simulink model "Monitoring_R2017b"  (R2017b)
settings: Solver=FixedStepAuto  StartTime=0.0  StopTime=inf  FixedStep=0.01  RelTol=1e-3
undefined symbols (not defined in the file): f
libraries: aerolibanimutils x1, instrumentlib x1
settings Model: Creator=guilherme  LastModifiedBy=leona

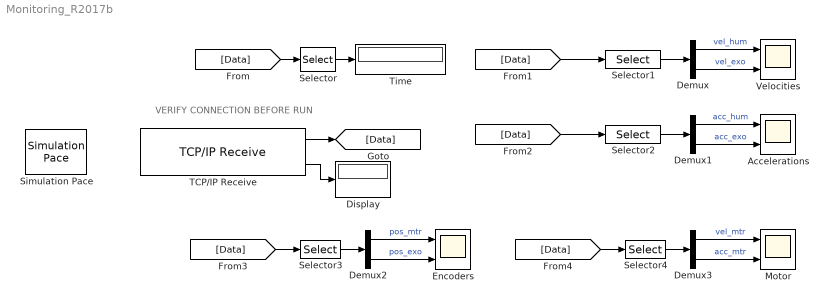
== system Monitoring_R2017b ==
  note: VERIFY CONNECTION BEFORE RUN
  Accelerations : Scope  NumInputPorts=2
  Demux{,1..3} (4 alike) : Demux  Outputs=2
  Display : Display
  Encoders : Scope  NumInputPorts=2
  Motor : Scope  NumInputPorts=2
  Selector : Selector  InputPortWidth=9  IndexOptions=Index vector (dialog)  Indices=[1]  OutputSizes=1
  Selector1 : Selector  InputPortWidth=9  IndexOptions=Index vector (dialog)  Indices=[2 3]  OutputSizes=1
  Selector2 : Selector  InputPortWidth=9  IndexOptions=Index vector (dialog)  Indices=[4 5]  OutputSizes=1
  Selector3 : Selector  InputPortWidth=9  IndexOptions=Index vector (dialog)  Indices=[6 7]  OutputSizes=1
  Selector4 : Selector  InputPortWidth=9  IndexOptions=Index vector (dialog)  Indices=[8 9]  OutputSizes=1
  Simulation Pace : aerolibanimutils/Simulation Pace  SimulationPace=1  SleepMode=Auto  OutputPaceError=off  SampleTime=-1
  TCP/IP Receive : instrumentlib/TCP//IP Receive  Host=0.0.0.0  Port=2324  DataSize="[1  9]"  EnableBlockingMode=off  Timeout=10  SampleTime=0.01  DataType=ASCII  ByteOrder=BigEndian  ASCIIFormatting=%f,%f,%f,%f,%f,%f,%f,%f,%f  Terminator=LF
  Time : Display
  Velocities : Scope  NumInputPorts=2
  wires:
  Selector/1 -> Time/1
  Demux/1 -> Velocities/1  "vel_hum"
  Demux/2 -> Velocities/2  "vel_exo"
  Selector1/1 -> Demux/1
  Selector2/1 -> Demux1/1
  Demux1/2 -> Accelerations/2  "acc_exo"
  Demux1/1 -> Accelerations/1  "acc_hum"
  Demux2/1 -> Encoders/1  "pos_mtr"
  Demux2/2 -> Encoders/2  "pos_exo"
  Selector3/1 -> Demux2/1
  TCP/IP Receive/1 -> [Data]
  [Data] -> Selector/1
  [Data] -> Selector1/1
  [Data] -> Selector2/1
  [Data] -> Selector3/1
  [Data] -> Selector4/1
  Selector4/1 -> Demux3/1
  Demux3/2 -> Motor/2  "acc_mtr"
  Demux3/1 -> Motor/1  "vel_mtr"
  TCP/IP Receive/2 -> Display/1
